simulink model "Transitions2"  (R2020a)
settings: Solver=VariableStepAuto  StartTime=0.0  StopTime=0.2  RelTol=1e-3
settings Model: Creator=BEAR  LastModifiedBy=bzhan
settings DataIOCC: ReturnWorkspaceOutputs=off
settings DebuggingCC: ArithmeticOperatorsInVariantConditions=warning
settings SFSimCC: SimUseLocalCustomCode=off  CustomCodeUndefinedFunction=UseInterfaceOnly
settings RTWCC: RTWUseLocalCustomCode=off

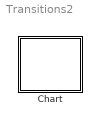
== system Transitions2 ==
  Chart : Stateflow chart  TreatAsAtomicUnit=on

== stateflow chart Transitions2/Chart ==
  settings: updateMethod=DISCRETE  sampleTime=0.1
  state S
    en: f("enS")
    ex: f("exS")
    state A
      en: f("enA")
      ex: f("exA")
    state B
      en: f("enB")
      ex: f("exB")
    (default) -> A
    A -> B
  state T
    en: f("enT")
    ex: f("exT")
    state C
      en: f("enB")
      ex: f("exB")
    (default) -> C
  (default) -> S
  B -> T : {f("ca")}/{f("ta")}
  data: s function_input
  function f(s):
    | function f(s)
    |   fprintf(s+"\n");
